simulink model "sim_tnse_2024_pos_ctrl"  (R2020a)
settings: Solver=ode4  StartTime=0.0  StopTime=30.0  FixedStep=0.01  RelTol=1e-3
values from neighbouring files (symbols this model uses):
  alfa_theta = 20    [init_tnse_2024_pos_ctrl.m]
  c1 = diag( [ 150.0, 120.0, 120.0 ] )    [init_tnse_2024_pos_ctrl.m]
  c1_diff_sigma_bar_v = diag([25; 30; 20])    [init_tnse_2024_pos_ctrl.m]
  c1v = diag([5.8; 6.5; 6.5])    [init_tnse_2024_pos_ctrl.m]
  c2 = diag( [ 80.0, 50.0, 50.0 ] )    [init_tnse_2024_pos_ctrl.m]
  c2_diff_sigma_bar_v = diag([50; 50; 10])    [init_tnse_2024_pos_ctrl.m]
  c2v = diag([5.8; 6.5; 6.5])    [init_tnse_2024_pos_ctrl.m]
  c3_diff_sigma_bar_v = diag([15; 15; 10])    [init_tnse_2024_pos_ctrl.m]
  c3v = diag([4.8; 6.4; 6.0])    [init_tnse_2024_pos_ctrl.m]
  dp_aa_t = 0.2 * ones(3, 5) + ( 1.0 - 0.2 ) * rand(3, 5)    [init_tnse_2024_pos_ctrl.m]
  dp_ff_t = [ 0.4 * ones(1, 5) + ( 1.0 - 0.4 ) * rand(1, 5);                      0.4 * ones(1, 5) + ( 1.0 - 0.4 ) * rand(1, 5);                      0.2 * ones(1, 5) + ( 0.6 - 0.2 ) * rand(1, 5) ]    [init_tnse_2024_pos_ctrl.m]
  dp_phi_t = ( - pi / 2 ) * ones(3, 5) + ( pi / 2 - ( - pi / 2 ) ) * rand(3, 5)    [init_tnse_2024_pos_ctrl.m]
  eps0 = [0.05; 0.01; 0.01]    [init_tnse_2024_pos_ctrl.m]
  etai_0 = zeros(3,5)    [init_tnse_2024_pos_ctrl.m]
  kai0 = [15; 10; 10]    [init_tnse_2024_pos_ctrl.m]
  kai_1_t = 0.02    [init_tnse_2024_pos_ctrl.m]
  kai_3_t = 0.1    [init_tnse_2024_pos_ctrl.m]
  ksii_0 = zeros(3,5)    [init_tnse_2024_pos_ctrl.m]
  lam0 = [15; 10; 10]    [init_tnse_2024_pos_ctrl.m]
  Lamd_diff_sigma_bar_v = 0.5    [init_tnse_2024_pos_ctrl.m]
  mass_i = zeros(1,NF)    [init_tnse_2024_pos_ctrl.m]
  Mii = diag([1;0;0;0;1])    [init_tnse_2024_pos_ctrl.m]
  pos0 = zeros(3, 1)    [init_tnse_2024_pos_ctrl.m]
  PZ0 = P0(3)    [init_tnse_2024_pos_ctrl.m]
  PZ1 = 10    [init_tnse_2024_pos_ctrl.m]
  Qci_init = repmat([1;0;0;0],1,NF)    [init_tnse_2024_pos_ctrl.m]
  R0 = 4    [init_tnse_2024_pos_ctrl.m]
  R1 = 8    [init_tnse_2024_pos_ctrl.m]
  Rx2 = 10    [init_tnse_2024_pos_ctrl.m]
  Ry2 = 6    [init_tnse_2024_pos_ctrl.m]
  Rz2 = 4    [init_tnse_2024_pos_ctrl.m]
  sat_sr_low = [-30, -30, -30]    [init_tnse_2024_pos_ctrl.m]
  sat_sr_up = [30, 30, 30]    [init_tnse_2024_pos_ctrl.m]
  T0 = 0    [init_tnse_2024_pos_ctrl.m]
  T1 = tseq1    (= 10)    [init_tnse_2024_pos_ctrl.m]
  T12 = tseq1 + tseq12    (= 20)    [init_tnse_2024_pos_ctrl.m]
  T2 = tseq1 + tseq12 + tseq2    (= 30)    [init_tnse_2024_pos_ctrl.m]
  theta0 = ( 2 / 5 ) * pi    (= 1.25663706144)    [init_tnse_2024_pos_ctrl.m]
  vel0 = zeros(3, 1)    [init_tnse_2024_pos_ctrl.m]
  Wij = [0,0,1,0,0;              0,0,1,1,0;              1,0,0,0,1;              0,1,1,0,0;              0,0,1,0,0]    [init_tnse_2024_pos_ctrl.m]
  X1 = 8    [init_tnse_2024_pos_ctrl.m]
  X2 = 2    [init_tnse_2024_pos_ctrl.m]
  X3 = 3    [init_tnse_2024_pos_ctrl.m]
  Y1 = 10    [init_tnse_2024_pos_ctrl.m]
  Y2 = 2    [init_tnse_2024_pos_ctrl.m]
  Y3 = 4    [init_tnse_2024_pos_ctrl.m]
  Z1 = 4    [init_tnse_2024_pos_ctrl.m]
  Z2 = -6    [init_tnse_2024_pos_ctrl.m]
  Z3 = 2    [init_tnse_2024_pos_ctrl.m]
  zeta_diff_sigma_bar_v = 0.08    [init_tnse_2024_pos_ctrl.m]
undefined symbols (not defined in the file or in its folder): cal_frac_squ, p_alfav1, p_alfav2, q_alfav1, q_alfav2
(part 4 of 4)

== matlab function sim_tnse_2024_pos_ctrl/follower tracking error agent 1 ==
  data: ksi_track_err_1 output; delta_ksi_vec input; delta_eta_vec input; ksi_i_vec input; eta_i_vec input; ksi0 input; eta_track_err_1 output; eta0 input
function [ksi_track_err_1, eta_track_err_1]  = fcn(delta_ksi_vec, delta_eta_vec, ksi_i_vec, eta_i_vec, ksi0, eta0)
%%%% 计算跟随者节点1号位置/速度跟踪误差
eta_track_err_1 = eta_i_vec(:,1) - delta_eta_vec(:,1) - eta0;
ksi_track_err_1 = ksi_i_vec(:,1) - delta_ksi_vec(:,1) - ksi0;

== matlab function sim_tnse_2024_pos_ctrl/follower tracking error agent 2 ==
  data: ksi_track_err_2 output; delta_ksi_vec input; delta_eta_vec input; ksi_i_vec input; eta_i_vec input; ksi0 input; eta_track_err_2 output; eta0 input
function [ksi_track_err_2, eta_track_err_2]  = fcn(delta_ksi_vec, delta_eta_vec, ksi_i_vec, eta_i_vec, ksi0, eta0)
%%%% 计算跟随者节点2号位置/速度跟踪误差
eta_track_err_2 = eta_i_vec(:,2) - delta_eta_vec(:,2) - eta0;
ksi_track_err_2 = ksi_i_vec(:,2) - delta_ksi_vec(:,2) - ksi0;

== matlab function sim_tnse_2024_pos_ctrl/follower tracking error agent 3 ==
  data: ksi_track_err_3 output; delta_ksi_vec input; delta_eta_vec input; ksi_i_vec input; eta_i_vec input; ksi0 input; eta_track_err_3 output; eta0 input
function [ksi_track_err_3, eta_track_err_3]  = fcn(delta_ksi_vec, delta_eta_vec, ksi_i_vec, eta_i_vec, ksi0, eta0)
%%%% 计算跟随者节点3号位置/速度跟踪误差
eta_track_err_3 = eta_i_vec(:,3) - delta_eta_vec(:,3) - eta0;
ksi_track_err_3 = ksi_i_vec(:,3) - delta_ksi_vec(:,3) - ksi0;

== matlab function sim_tnse_2024_pos_ctrl/follower tracking error agent 4 ==
  data: ksi_track_err_4 output; delta_ksi_vec input; delta_eta_vec input; ksi_i_vec input; eta_i_vec input; ksi0 input; eta_track_err_4 output; eta0 input
function [ksi_track_err_4, eta_track_err_4]  = fcn(delta_ksi_vec, delta_eta_vec, ksi_i_vec, eta_i_vec, ksi0, eta0)
%%%% 计算跟随者节点4号位置/速度跟踪误差
eta_track_err_4 = eta_i_vec(:,4) - delta_eta_vec(:,4) - eta0;
ksi_track_err_4 = ksi_i_vec(:,4) - delta_ksi_vec(:,4) - ksi0;

== matlab function sim_tnse_2024_pos_ctrl/follower tracking error agent 5 ==
  data: ksi_track_err_5 output; delta_ksi_vec input; delta_eta_vec input; ksi_i_vec input; eta_i_vec input; ksi0 input; eta_track_err_5 output; eta0 input
function [ksi_track_err_5, eta_track_err_5]  = fcn(delta_ksi_vec, delta_eta_vec, ksi_i_vec, eta_i_vec, ksi0, eta0)
%%%% 计算跟随者节点5号位置/速度跟踪误差
eta_track_err_5 = eta_i_vec(:,5) - delta_eta_vec(:,5) - eta0;
ksi_track_err_5 = ksi_i_vec(:,5) - delta_ksi_vec(:,5) - ksi0;

== matlab function sim_tnse_2024_pos_ctrl/combine follower eta ksi ==
  data: ksi_track_err_vec output; ksi_track_err_1 input; ksi_track_err_2 input; ksi_track_err_3 input; ksi_track_err_4 input; ksi_track_err_5 input; eta_track_err_vec output; eta_track_err_1 input; eta_track_err_2 input; eta_track_err_3 input; eta_track_err_4 input; eta_track_err_5 input
function [ksi_track_err_vec, eta_track_err_vec]  = fcn(ksi_track_err_1, ksi_track_err_2, ksi_track_err_3, ksi_track_err_4, ksi_track_err_5, ...
                                                                                    eta_track_err_1, eta_track_err_2, eta_track_err_3, eta_track_err_4, eta_track_err_5)
%%%% 合并所有跟随者的速度/位置向量
ksi_track_err_vec = [ksi_track_err_1(:), ksi_track_err_2(:), ksi_track_err_3(:), ksi_track_err_4(:), ksi_track_err_5(:)];
eta_track_err_vec = [eta_track_err_1(:), eta_track_err_2(:), eta_track_err_3(:), eta_track_err_4(:), eta_track_err_5(:)];

== matlab function sim_tnse_2024_pos_ctrl/depart Rc5 ==
  data: y output; x input
function y = fcn(x)
y = x(:,:,5);

end

== matlab function sim_tnse_2024_pos_ctrl/depart Rc1 ==
  data: y output; x input
function y = fcn(x)
y = x(:,:,1);

end

== matlab function sim_tnse_2024_pos_ctrl/depart Rc2 ==
  data: y output; x input
function y = fcn(x)
y = x(:,:,2);

end

== matlab function sim_tnse_2024_pos_ctrl/depart Rc3 ==
  data: y output; x input
function y = fcn(x)
y = x(:,:,3);

end

== matlab function sim_tnse_2024_pos_ctrl/depart Rc4 ==
  data: y output; x input
function y = fcn(x)
y = x(:,:,4);

end

== matlab function sim_tnse_2024_pos_ctrl/combine rho_hat ==
  data: rho_hat_1 input; rho_hat_vec output; rho_hat_2 input; rho_hat_3 input; rho_hat_4 input; rho_hat_5 input
function rho_hat_vec  = fcn(rho_hat_1, rho_hat_2, rho_hat_3, rho_hat_4, rho_hat_5)
%%%% 合并领导者加速度分布式观测器
rho_hat_vec = zeros(3,5);
rho_hat_vec(:,1) = rho_hat_1(:);
rho_hat_vec(:,2) = rho_hat_2(:);
rho_hat_vec(:,3) = rho_hat_3(:);
rho_hat_vec(:,4) = rho_hat_4(:);
rho_hat_vec(:,5) = rho_hat_5(:);

== matlab function sim_tnse_2024_pos_ctrl/rho_hat agent 1 ==
  data: lam0 input; rho_hat_1 output; sigmai_vec input
function rho_hat_1 = fcn(lam0, sigmai_vec)
%%%% 领导者加速度分布式观测器
iiuav = 1;
rho_hat_1 = lam0(:) .* tanh( sigmai_vec(:,iiuav) );

== matlab function sim_tnse_2024_pos_ctrl/rho_hat agent 2 ==
  data: lam0 input; rho_hat_2 output; sigmai_vec input
function rho_hat_2 = fcn(lam0, sigmai_vec)
%%%% 领导者加速度分布式观测器
iiuav = 2;
rho_hat_2 = lam0(:) .* tanh( sigmai_vec(:,iiuav) );

== matlab function sim_tnse_2024_pos_ctrl/rho_hat agent 3 ==
  data: lam0 input; rho_hat_3 output; sigmai_vec input
function rho_hat_3 = fcn(lam0, sigmai_vec)
%%%% 领导者加速度分布式观测器
iiuav = 3;
rho_hat_3 = lam0(:) .* tanh( sigmai_vec(:,iiuav) );

== matlab function sim_tnse_2024_pos_ctrl/rho_hat agent 4 ==
  data: lam0 input; rho_hat_4 output; sigmai_vec input
function rho_hat_4 = fcn(lam0, sigmai_vec)
%%%% 领导者加速度分布式观测器
iiuav = 4;
rho_hat_4 = lam0(:) .* tanh( sigmai_vec(:,iiuav) );

== matlab function sim_tnse_2024_pos_ctrl/rho_hat agent 5 ==
  data: lam0 input; rho_hat_5 output; sigmai_vec input
function rho_hat_5 = fcn(lam0, sigmai_vec)
%%%% 领导者加速度分布式观测器
iiuav = 5;
rho_hat_5 = lam0(:) .* tanh( sigmai_vec(:,iiuav) );

== matlab function sim_tnse_2024_pos_ctrl/cal si agent 1 ==
  data: Wij input; Mii input; si_1 output; delta_ksi_vec input; ksi0 input; ksi_i_vec input; ksi_d_est_vec input
function si_1 = fcn(Wij, Mii, delta_ksi_vec, ksi0, ksi_i_vec, ksi_d_est_vec)
%%%% 计算位置误差面
iiuav = 1;
si_1 = Mii(iiuav, iiuav) * ( ksi_i_vec(:,iiuav) - ksi0(:) - delta_ksi_vec(:,iiuav) ) ...
            + Mii(iiuav, iiuav) * ( ksi_d_est_vec(:,iiuav) - ksi0(:) );
for jjuav = 1:5
    si_1 = si_1 + Wij(iiuav, jjuav) * ( ( ksi_i_vec(:,iiuav) - delta_ksi_vec(:,iiuav) ) - ( ksi_i_vec(:,jjuav) - delta_ksi_vec(:,jjuav) ) ) ...
                        + Wij(iiuav, jjuav) * ( ksi_d_est_vec(:,iiuav) - ksi_d_est_vec(:,jjuav) );
end

== matlab function sim_tnse_2024_pos_ctrl/generate translational disturbance agent 1 ==
  data: dp_aa_t input; dp_ff_t input; dp_phi_t input; dp_1 output; t input
function dp_1 = fcn(dp_aa_t, dp_ff_t, dp_phi_t, t)
%%%% 平移动力学方程中的扰动项设置
epsil_t = zeros(3, 1);

for kk = 1:5
    epsil_t = epsil_t + dp_aa_t(:, kk) .* sin( 2 * pi * dp_ff_t(:, kk) * t + dp_phi_t(:, kk) );
end

dp_1 = [ epsil_t(1) + 1.6 * sin( 0.4 * t ) + 2.0 * cos( 0.5 * t ) + 1.4 * sin( 0.7 * t ) ...
                + 4 * exp( -0.1 * t ) * sin( 0.8 * t ) + 3 / ( 1 + exp( -0.2 * ( t - 15 ) ) ); ...
                epsil_t(2) + 1.2 * sin( 0.2 * t ) + 3 * cos( 0.4 * t ) + 0.8 * sin( 0.6 * t ) ...
                + 2 * exp( -0.15 * t ) * cos( 1.2 * t ) + 3 / ( 1 + exp( -0.3 * ( t - 25 ) ) ); ...
                epsil_t(3) + 1.8 * sin( 0.2 * t ) + 1.6 * sin( 0.3 * t ) + 1.6 * cos( 0.4 * t ) ...
                + 4 * exp( -0.05 * t ) * sin( 0.5 * t + pi / 4 ) + 3 / ( 1 + exp( -0.5 * ( t - 20 ) ) ) ];

== matlab function sim_tnse_2024_pos_ctrl/update dpsy psy agent 1 ==
  data: Wij input; Mii input; d_2_psy_1 output; delta_ksi_vec input; delta_eta_vec input; ksi_i_vec input; eta_i_vec input; ksi_d_est_vec input; eta_d_est_vec input
function d_2_psy_1 = fcn(Wij, Mii, delta_ksi_vec, delta_eta_vec, ksi_i_vec, eta_i_vec, ksi_d_est_vec, eta_d_est_vec)
%%%% 计算集群构型估计二阶导数
iiuav = 1;
err_v_est = Mii(iiuav, iiuav) * ( eta_d_est_vec(:,iiuav) - ( eta_i_vec(:,iiuav) - delta_eta_vec(:,iiuav) ) );
err_p_est = Mii(iiuav, iiuav) * ( ksi_d_est_vec(:,iiuav) - ( ksi_i_vec(:,iiuav) - delta_ksi_vec(:,iiuav) ) );
for jjuav = 1:5
    err_v_est = err_v_est + Wij(iiuav, jjuav) * ( ( eta_d_est_vec(:,iiuav) - ( eta_i_vec(:,iiuav) - delta_eta_vec(:,iiuav) ) ) ...
                                                                                - ( eta_d_est_vec(:,jjuav) - ( eta_i_vec(:,jjuav) - delta_eta_vec(:,jjuav) ) ) );
    err_p_est = err_p_est + Wij(iiuav, jjuav) * ( ( ksi_d_est_vec(:,iiuav) - ( ksi_i_vec(:,iiuav) - delta_ksi_vec(:,iiuav) ) ) ...
                                                                                - ( ksi_d_est_vec(:,jjuav) - ( ksi_i_vec(:,jjuav) - delta_ksi_vec(:,jjuav) ) ) );
end
d_2_psy_1 = -err_v_est(:) - err_p_est(:);

== matlab function sim_tnse_2024_pos_ctrl/cal si agent 3 ==
  data: Wij input; Mii input; si_3 output; delta_ksi_vec input; ksi0 input; ksi_i_vec input; ksi_d_est_vec input
function si_3 = fcn(Wij, Mii, delta_ksi_vec, ksi0, ksi_i_vec, ksi_d_est_vec)
%%%% 计算位置误差面
iiuav = 3;
si_3 = Mii(iiuav, iiuav) * ( ksi_i_vec(:,iiuav) - ksi0(:) - delta_ksi_vec(:,iiuav) ) ...
            + Mii(iiuav, iiuav) * ( ksi_d_est_vec(:,iiuav) - ksi0(:) );
for jjuav = 1:5
    si_3 = si_3 + Wij(iiuav, jjuav) * ( ( ksi_i_vec(:,iiuav) - delta_ksi_vec(:,iiuav) ) - ( ksi_i_vec(:,jjuav) - delta_ksi_vec(:,jjuav) ) ) ...
                        + Wij(iiuav, jjuav) * ( ksi_d_est_vec(:,iiuav) - ksi_d_est_vec(:,jjuav) );
end

== matlab function sim_tnse_2024_pos_ctrl/cal si agent 4 ==
  data: Wij input; Mii input; si_4 output; delta_ksi_vec input; ksi0 input; ksi_i_vec input; ksi_d_est_vec input
function si_4 = fcn(Wij, Mii, delta_ksi_vec, ksi0, ksi_i_vec, ksi_d_est_vec)
%%%% 计算位置误差面
iiuav = 4;
si_4 = Mii(iiuav, iiuav) * ( ksi_i_vec(:,iiuav) - ksi0(:) - delta_ksi_vec(:,iiuav) ) ...
            + Mii(iiuav, iiuav) * ( ksi_d_est_vec(:,iiuav) - ksi0(:) );
for jjuav = 1:5
    si_4 = si_4 + Wij(iiuav, jjuav) * ( ( ksi_i_vec(:,iiuav) - delta_ksi_vec(:,iiuav) ) - ( ksi_i_vec(:,jjuav) - delta_ksi_vec(:,jjuav) ) ) ...
                        + Wij(iiuav, jjuav) * ( ksi_d_est_vec(:,iiuav) - ksi_d_est_vec(:,jjuav) );
end

== matlab function sim_tnse_2024_pos_ctrl/cal si agent 5 ==
  data: Wij input; Mii input; si_5 output; delta_ksi_vec input; ksi0 input; ksi_i_vec input; ksi_d_est_vec input
function si_5 = fcn(Wij, Mii, delta_ksi_vec, ksi0, ksi_i_vec, ksi_d_est_vec)
%%%% 计算位置误差面
iiuav = 5;
si_5 = Mii(iiuav, iiuav) * ( ksi_i_vec(:,iiuav) - ksi0(:) - delta_ksi_vec(:,iiuav) ) ...
            + Mii(iiuav, iiuav) * ( ksi_d_est_vec(:,iiuav) - ksi0(:) );
for jjuav = 1:5
    si_5 = si_5 + Wij(iiuav, jjuav) * ( ( ksi_i_vec(:,iiuav) - delta_ksi_vec(:,iiuav) ) - ( ksi_i_vec(:,jjuav) - delta_ksi_vec(:,jjuav) ) ) ...
                        + Wij(iiuav, jjuav) * ( ksi_d_est_vec(:,iiuav) - ksi_d_est_vec(:,jjuav) );
end

== matlab function sim_tnse_2024_pos_ctrl/cal ri agent 2 ==
  data: Wij input; Mii input; delta_eta_vec input; ri_2 output; eta0 input; eta_i_vec input; eta_d_est_vec input
function ri_2 = fcn(Wij, Mii, delta_eta_vec, eta0, eta_i_vec, eta_d_est_vec)
%%%% 计算速度误差面
iiuav = 2;
ri_2 = Mii(iiuav, iiuav) * ( eta_i_vec(:,iiuav) - eta0(:) - delta_eta_vec(:,iiuav) ) ...
            + Mii(iiuav, iiuav) * ( eta_d_est_vec(:,iiuav) - eta0(:) );
for jjuav = 1:5
    ri_2 = ri_2 + Wij(iiuav, jjuav) * ( ( eta_i_vec(:,iiuav) - delta_eta_vec(:,iiuav) ) - ( eta_i_vec(:,jjuav) - delta_eta_vec(:,jjuav) ) ) ...
                        + Wij(iiuav, jjuav) * ( eta_d_est_vec(:,iiuav) - eta_d_est_vec(:,jjuav) );
end

== matlab function sim_tnse_2024_pos_ctrl/combine d_psy ==
  data: d_psy_1 input; d_psy_2 input; d_psy_3 input; d_psy_4 input; d_psy_5 input; d_psy_vec output
function d_psy_vec  = fcn(d_psy_1, d_psy_2, d_psy_3, d_psy_4, d_psy_5)
%%%% 合并集群构型估计导数
d_psy_vec = zeros(3,5);
d_psy_vec(:,1) = d_psy_1(:);
d_psy_vec(:,2) = d_psy_2(:);
d_psy_vec(:,3) = d_psy_3(:);
d_psy_vec(:,4) = d_psy_4(:);
d_psy_vec(:,5) = d_psy_5(:);

== matlab function sim_tnse_2024_pos_ctrl/combine psy ==
  data: psy_1 input; psy_2 input; psy_3 input; psy_4 input; psy_5 input; psy_vec output
function psy_vec  = fcn(psy_1, psy_2, psy_3, psy_4, psy_5)
%%%% 合并集群构型估计量
psy_vec = zeros(3,5);
psy_vec(:,1) = psy_1(:);
psy_vec(:,2) = psy_2(:);
psy_vec(:,3) = psy_3(:);
psy_vec(:,4) = psy_4(:);
psy_vec(:,5) = psy_5(:);

== matlab function sim_tnse_2024_pos_ctrl/cal eta_d_est ksi_d_est ==
  data: d_psy_vec input; psy_vec input; eta_d_est_vec output; eta_i_vec input; ksi_i_vec input; ksi_d_est_vec output
function [eta_d_est_vec, ksi_d_est_vec] = fcn(d_psy_vec, psy_vec, eta_i_vec, ksi_i_vec)
%%%% 计算跟随者期望速度/位置
eta_d_est_vec = zeros(3,5);
ksi_d_est_vec = zeros(3,5);
for iiuav = 1:5
    eta_d_est_vec(:,iiuav) = eta_i_vec(:,iiuav) + d_psy_vec(:,iiuav);
    ksi_d_est_vec(:,iiuav) = ksi_i_vec(:,iiuav) + psy_vec(:,iiuav);
end

== matlab function sim_tnse_2024_pos_ctrl/generate translational disturbance agent 2 ==
  data: dp_aa_t input; dp_ff_t input; dp_phi_t input; dp_2 output; t input
function dp_2 = fcn(dp_aa_t, dp_ff_t, dp_phi_t, t)
%%%% 平移动力学方程中的扰动项设置
epsil_t = zeros(3, 1);

for kk = 1:5
    epsil_t = epsil_t + dp_aa_t(:, kk) .* sin( 2 * pi * dp_ff_t(:, kk) * t + dp_phi_t(:, kk) );
end

dp_2 = [ epsil_t(1) + 1.6 * sin( 0.2 * t ) + 2.0 * cos( 0.3 * t ) + 1.4 * sin( 0.5 * t ) ...
                + 4 * exp( -0.1 * t ) * sin( 0.5 * t ) + 3 / ( 1 + exp( -0.2 * ( t - 15 ) ) ); ...
                epsil_t(2) + 1.2 * sin( 0.1 * t ) + 3 * cos( 0.2 * t ) + 0.8 * sin( 0.4 * t ) ...
                + 2 * exp( -0.15 * t ) * cos( 0.6 * t ) + 3 / ( 1 + exp( -0.3 * ( t - 25 ) ) ); ...
                epsil_t(3) + 1.8 * sin( 0.1 * t ) + 1.6 * sin( 0.2 * t ) + 1.6 * cos( 0.3 * t ) ...
                + 4 * exp( -0.05 * t ) * sin( 0.4 * t + pi / 4 ) + 3 / ( 1 + exp( -0.5 * ( t - 20 ) ) ) ];

== matlab function sim_tnse_2024_pos_ctrl/cal ri agent 3 ==
  data: Wij input; Mii input; delta_eta_vec input; ri_3 output; eta0 input; eta_i_vec input; eta_d_est_vec input
function ri_3 = fcn(Wij, Mii, delta_eta_vec, eta0, eta_i_vec, eta_d_est_vec)
%%%% 计算速度误差面
iiuav = 3;
ri_3 = Mii(iiuav, iiuav) * ( eta_i_vec(:,iiuav) - eta0(:) - delta_eta_vec(:,iiuav) ) ...
            + Mii(iiuav, iiuav) * ( eta_d_est_vec(:,iiuav) - eta0(:) );
for jjuav = 1:5
    ri_3 = ri_3 + Wij(iiuav, jjuav) * ( ( eta_i_vec(:,iiuav) - delta_eta_vec(:,iiuav) ) - ( eta_i_vec(:,jjuav) - delta_eta_vec(:,jjuav) ) ) ...
                        + Wij(iiuav, jjuav) * ( eta_d_est_vec(:,iiuav) - eta_d_est_vec(:,jjuav) );
end

== matlab function sim_tnse_2024_pos_ctrl/cal ri agent 4 ==
  data: Wij input; Mii input; delta_eta_vec input; ri_4 output; eta0 input; eta_i_vec input; eta_d_est_vec input
function ri_4 = fcn(Wij, Mii, delta_eta_vec, eta0, eta_i_vec, eta_d_est_vec)
%%%% 计算速度误差面
iiuav = 4;
ri_4 = Mii(iiuav, iiuav) * ( eta_i_vec(:,iiuav) - eta0(:) - delta_eta_vec(:,iiuav) ) ...
            + Mii(iiuav, iiuav) * ( eta_d_est_vec(:,iiuav) - eta0(:) );
for jjuav = 1:5
    ri_4 = ri_4 + Wij(iiuav, jjuav) * ( ( eta_i_vec(:,iiuav) - delta_eta_vec(:,iiuav) ) - ( eta_i_vec(:,jjuav) - delta_eta_vec(:,jjuav) ) ) ...
                        + Wij(iiuav, jjuav) * ( eta_d_est_vec(:,iiuav) - eta_d_est_vec(:,jjuav) );
end

== matlab function sim_tnse_2024_pos_ctrl/cal ri agent 5 ==
  data: Wij input; Mii input; delta_eta_vec input; ri_5 output; eta0 input; eta_i_vec input; eta_d_est_vec input
function ri_5 = fcn(Wij, Mii, delta_eta_vec, eta0, eta_i_vec, eta_d_est_vec)
%%%% 计算速度误差面
iiuav = 5;
ri_5 = Mii(iiuav, iiuav) * ( eta_i_vec(:,iiuav) - eta0(:) - delta_eta_vec(:,iiuav) ) ...
            + Mii(iiuav, iiuav) * ( eta_d_est_vec(:,iiuav) - eta0(:) );
for jjuav = 1:5
    ri_5 = ri_5 + Wij(iiuav, jjuav) * ( ( eta_i_vec(:,iiuav) - delta_eta_vec(:,iiuav) ) - ( eta_i_vec(:,jjuav) - delta_eta_vec(:,jjuav) ) ) ...
                        + Wij(iiuav, jjuav) * ( eta_d_est_vec(:,iiuav) - eta_d_est_vec(:,jjuav) );
end

== matlab function sim_tnse_2024_pos_ctrl/combine si ==
  data: si_1 input; si_2 input; si_3 input; si_4 input; si_5 input; si_vec output
function si_vec  = fcn(si_1, si_2, si_3, si_4, si_5)
%%%% 合并位置跟踪误差
si_vec = zeros(3,5);
si_vec(:,1) = si_1(:);
si_vec(:,2) = si_2(:);
si_vec(:,3) = si_3(:);
si_vec(:,4) = si_4(:);
si_vec(:,5) = si_5(:);

== matlab function sim_tnse_2024_pos_ctrl/cal ri agent 1 ==
  data: Wij input; Mii input; delta_eta_vec input; ri_1 output; eta0 input; eta_i_vec input; eta_d_est_vec input
function ri_1 = fcn(Wij, Mii, delta_eta_vec, eta0, eta_i_vec, eta_d_est_vec)
%%%% 计算速度误差面
iiuav = 1;
ri_1 = Mii(iiuav, iiuav) * ( eta_i_vec(:,iiuav) - eta0(:) - delta_eta_vec(:,iiuav) ) ...
            + Mii(iiuav, iiuav) * ( eta_d_est_vec(:,iiuav) - eta0(:) );
for jjuav = 1:5
    ri_1 = ri_1 + Wij(iiuav, jjuav) * ( ( eta_i_vec(:,iiuav) - delta_eta_vec(:,iiuav) ) - ( eta_i_vec(:,jjuav) - delta_eta_vec(:,jjuav) ) ) ...
                        + Wij(iiuav, jjuav) * ( eta_d_est_vec(:,iiuav) - eta_d_est_vec(:,jjuav) );
end

== matlab function sim_tnse_2024_pos_ctrl/combine ri ==
  data: ri_1 input; ri_2 input; ri_3 input; ri_4 input; ri_5 input; ri_vec output
function ri_vec  = fcn(ri_1, ri_2, ri_3, ri_4, ri_5)
%%%% 合并速度跟踪误差
ri_vec = zeros(3,5);
ri_vec(:,1) = ri_1(:);
ri_vec(:,2) = ri_2(:);
ri_vec(:,3) = ri_3(:);
ri_vec(:,4) = ri_4(:);
ri_vec(:,5) = ri_5(:);

== matlab function sim_tnse_2024_pos_ctrl/leader control input ==
  data: t input; u0 output; T1 input; T2 input; R0 input; R1 input; Rx2 input; Ry2 input; Rz2 input
function u0  = fcn(t, T1, T2, R0, R1, Rx2, Ry2, Rz2)
%%%% 给出领导者参考加速度控制输入
u0 = zeros(3, 1);

if t <= ( T1 + 1e-05 )
    u0(1, 1) = - ( 4 * pi * sin( ( 2 * pi * ( t - 0 ) ) / ( 0 - T1 ) ) * ( R0 - R1 ) ) / ( ( 0 - T1 ) ^ 2 ) ...
                        - ( 4 * ( pi ^ 2 ) * cos( ( 2 * pi * ( t - 0 ) ) / ( 0 - T1 ) ) ...
                        * ( R0 + ( ( R0 - R1 ) * ( t - 0 ) ) / ( 0 - T1 ) ) ) / ( ( 0 - T1 ) ^ 2 );
    u0(2, 1) = ( 4 * pi * cos( ( 2 * pi * ( t - 0 ) ) / ( 0 - T1 ) ) * ( R0 - R1 ) ) / ( ( 0 - T1 ) ^ 2 ) ...
                        - ( 4 * ( pi ^ 2 ) * sin( ( 2 * pi * ( t - 0 ) ) / ( 0 - T1 ) ) ...
                        * ( R0 + ( ( R0 - R1 ) * ( t - 0 ) ) / ( 0 - T1 ) ) ) / ( ( 0 - T1 ) ^ 2 );
    u0(3, 1) = 0;
else
    u0(1, 1) = ( 4 * Rx2 * ( pi ^ 2 ) * cos( ( 2 * pi * ( t - T1 ) ) / ( T1 - T2 ) ) ) / ( ( T1 - T2 ) ^ 2 );
    u0(2, 1) = - ( 16 * Ry2 * ( pi ^ 2 ) * sin( ( 4 * pi * ( t - T1 ) ) / ( T1 - T2 ) ) ) / ( ( T1 - T2 ) ^ 2 );
    u0(3, 1) = ( 16 * Rz2 * ( pi ^ 2 ) * sin( ( 4 * pi * ( t - T1 ) ) / ( T1 - T2 ) ) ) / ( ( T1 - T2 ) ^ 2 );
end

== matlab function sim_tnse_2024_pos_ctrl/process velocity ==
  data: T0 input; T1 input; T2 input; PZ0 input; PZ1 input; R0 input; R1 input; Rx2 input; Ry2 input; Rz2 input; t input; V_init_out output
function V_init_out = fcn(T0, T1, T2, PZ0, PZ1, R0, R1, Rx2, Ry2, Rz2, t)
V_init_out = zeros(3, 1);
if t < T1 + 1e-05
    V_init_out(1, 1) = ( cos( ( 2 * pi * ( t - T0 ) ) / ( T0 - T1 ) ) * ( R0 - R1 ) ) / ( T0 - T1 ) ...
                                    - ( 2 * pi * sin( ( 2 * pi * ( t - T0 ) ) / ( T0 - T1 ) ) * ( R0 + ( ( R0 - R1 ) * ( t - T0 ) ) / ( T0 - T1 ) ) ) / ( T0 - T1 );
    V_init_out(2, 1) = ( sin( ( 2 * pi * ( t - T0 ) ) / ( T0 - T1 ) ) * ( R0 - R1 ) ) / ( T0 - T1 ) ...
                                    + ( 2 * pi * cos( ( 2 * pi * ( t - T0 ) ) / ( T0 - T1 ) ) * ( R0 + ( ( R0 - R1 ) * ( t - T0 ) ) / ( T0 - T1 ) ) ) / ( T0 - T1 );
    V_init_out(3, 1) = ( PZ0 - PZ1 ) / ( T0 - T1 );
else
    V_init_out(1, 1) = ( 2 * Rx2 * pi * sin( ( 2 * pi * ( t - T1 ) ) / ( T1 - T2 ) ) ) / ( T1 - T2 );
    V_init_out(2, 1) = ( 4 * Ry2 * pi * cos( ( 4 * pi * ( t - T1 ) ) / ( T1 - T2 ) ) ) / ( T1 - T2 );
    V_init_out(3, 1) = - ( 4 * Rz2 * pi * cos( ( 4 * pi * ( t - T1 ) ) / ( T1 - T2 ) ) ) / ( T1 - T2 );
end

== matlab function sim_tnse_2024_pos_ctrl/generate translational disturbance agent 3 ==
  data: dp_aa_t input; dp_ff_t input; dp_phi_t input; dp_3 output; t input
function dp_3 = fcn(dp_aa_t, dp_ff_t, dp_phi_t, t)
%%%% 平移动力学方程中的扰动项设置
epsil_t = zeros(3, 1);

for kk = 1:5
    epsil_t = epsil_t + dp_aa_t(:, kk) .* sin( 2 * pi * dp_ff_t(:, kk) * t + dp_phi_t(:, kk) );
end

dp_3 = [ epsil_t(1) + 1.6 * sin( 0.2 * t ) + 2.0 * cos( 0.3 * t ) + 1.4 * sin( 0.5 * t ) ...
                + 4 * exp( -0.1 * t ) * sin( 0.5 * t ) + 3 / ( 1 + exp( -0.2 * ( t - 15 ) ) ); ...
                epsil_t(2) + 1.2 * sin( 0.1 * t ) + 3 * cos( 0.2 * t ) + 0.8 * sin( 0.4 * t ) ...
                + 2 * exp( -0.15 * t ) * cos( 0.6 * t ) + 3 / ( 1 + exp( -0.3 * ( t - 25 ) ) ); ...
                epsil_t(3) + 1.8 * sin( 0.1 * t ) + 1.6 * sin( 0.2 * t ) + 1.6 * cos( 0.3 * t ) ...
                + 4 * exp( -0.05 * t ) * sin( 0.4 * t + pi / 4 ) + 3 / ( 1 + exp( -0.5 * ( t - 20 ) ) ) ];

== matlab function sim_tnse_2024_pos_ctrl/set desire formation configuration ==
  data: X1 input; X2 input; X3 input; Y1 input; Y2 input; Y3 input; Z1 input; Z2 input; Z3 input; theta0 input; kai_1_t input; kai_3_t input; T1 input; T12 input; t input; delta_ksi_vec output; delta_eta_vec output; d_delta_eta_vec output
function [delta_ksi_vec, delta_eta_vec, d_delta_eta_vec] = fcn(X1, X2, X3, Y1, Y2, Y3, Z1, Z2, Z3, ...
                                                                                                                theta0, kai_1_t, kai_3_t, T1, T12, t)
%%%% 计算跟随者期望速度分布式观测器误差
delta_ksi_vec = zeros(3, 5);
delta_eta_vec = zeros(3, 5);
d_delta_eta_vec = zeros(3, 5);
if t <= ( T1 + 1e-04 )
    exp_tmp = exp( -kai_1_t * t );
    delta_ksi_vec(:, 1) = [ X1 * cos( theta0 ) - X2 * exp_tmp; ...
                                            Y1 * sin( theta0 ) - Y2 * exp_tmp; ...
                                            Z1 - Z2 * exp_tmp ];
    delta_ksi_vec(:, 2) = [ - X1 * cos( theta0 ) + X2 * exp_tmp; ...
                                            Y1 * sin( theta0 ) - Y2 * exp_tmp; ...
                                            Z1 + Z2 * exp_tmp ];
    delta_ksi_vec(:, 3) = [ X1 - X2 * exp_tmp; ...
                                            Y2 * exp_tmp; ...
                                            ( 3 / 8 ) * Z1 + Z2 * exp_tmp ];
    delta_ksi_vec(:, 4) = [ - X1 * cos( theta0 ) + X2 * exp_tmp; ...
                                            - Y1 * sin( theta0 ) + Y2 * exp_tmp; ...
                                            Z1 + Z2 * exp_tmp ];
    delta_ksi_vec(:, 5) = [ X1 * cos( theta0 ) - X2 * exp_tmp; ...
                                            - Y1 * sin( theta0 ) + Y2 * exp_tmp; ...
                                            Z1 - Z2 * exp_tmp ];
    delta_eta_vec(:, 1) = [ kai_1_t * X2 * exp_tmp; kai_1_t * Y2 * exp_tmp; kai_1_t * Z2 * exp_tmp ];
    delta_eta_vec(:, 2) = [ - kai_1_t * X2 * exp_tmp; kai_1_t * Y2 * exp_tmp; - kai_1_t * Z2 * exp_tmp ];
    delta_eta_vec(:, 3) = [ kai_1_t * X2 * exp_tmp; - kai_1_t * Y2 * exp_tmp; - kai_1_t * Z2 * exp_tmp ];
    delta_eta_vec(:, 4) = [ - kai_1_t * X2 * exp_tmp; - kai_1_t * Y2 * exp_tmp; - kai_1_t * Z2 * exp_tmp ];
    delta_eta_vec(:, 5) = [ kai_1_t * X2 * exp_tmp; - kai_1_t * Y2 * exp_tmp; kai_1_t * Z2 * exp_tmp ];
    d_delta_eta_vec(:, 1) = [ - ( kai_1_t ^ 2 ) * X2 * exp_tmp; - ( kai_1_t ^ 2 ) * Y2 * exp_tmp; - ( kai_1_t ^ 2 ) * Z2 * exp_tmp ];
    d_delta_eta_vec(:, 2) = [ ( kai_1_t ^ 2 ) * X2 * exp_tmp; - ( kai_1_t ^ 2 ) * Y2 * exp_tmp; ( kai_1_t ^ 2 ) * Z2 * exp_tmp ];
    d_delta_eta_vec(:, 3) = [ - ( kai_1_t ^ 2 ) * X2 * exp_tmp; ( kai_1_t ^ 2 ) * Y2 * exp_tmp; ( kai_1_t ^ 2 ) * Z2 * exp_tmp ];
    d_delta_eta_vec(:, 4) = [ ( kai_1_t ^ 2 ) * X2 * exp_tmp; ( kai_1_t ^ 2 ) * Y2 * exp_tmp; ( kai_1_t ^ 2 ) * Z2 * exp_tmp ];
    d_delta_eta_vec(:, 5) = [ - ( kai_1_t ^ 2 ) * X2 * exp_tmp; ( kai_1_t ^ 2 ) * Y2 * exp_tmp; - ( kai_1_t ^ 2 ) * Z2 * exp_tmp ];
elseif t <= ( T12 + 1e-04 )
    delta_ksi_vec(:, 1) = [ X1 * cos( theta0 ) - X2; Y1 * sin( theta0 ) - Y2; Z1 - Z2 ];
    delta_ksi_vec(:, 2) = [ - X1 * cos( theta0 ) + X2; Y1 * sin( theta0 ) - Y2; Z1 + Z2 ];
    delta_ksi_vec(:, 3) = [ X1 - X2; 0; ( 3 / 8 ) * Z1 + Z2 ];
    delta_ksi_vec(:, 4) = [ - X1 * cos( theta0 ) + X2; - Y1 * sin( theta0 ) + Y2; Z1 + Z2 ];
    delta_ksi_vec(:, 5) = [ X1 * cos( theta0 ) - X2; - Y1 * sin( theta0 ) + Y2; Z1 - Z2 ];
else
    exp_tmp = 1 / ( 1 + exp( - kai_3_t * ( t - T12 - 5 ) ) );
    tmp_2 = exp( - kai_3_t * ( t - T12 - 5 ) ) / ( ( 1 + exp( - kai_3_t * ( t - T12 - 5 ) ) ) ^ 2 );
    delta_ksi_vec(:, 1) = [ X1 * cos( theta0 ) - X2 + X3 * exp_tmp; ...
                                            Y1 * sin( theta0 ) - Y2 + Y3 * exp_tmp; ...
                                            Z1 - Z2 + Z3 * exp_tmp ];
    delta_ksi_vec(:, 2) = [ - X1 * cos( theta0 ) + X2 - X3 * exp_tmp; ...
                                            Y1 * sin( theta0 ) - Y2 + Y3 * exp_tmp; ...
                                            Z1 + Z2 - Z3 * exp_tmp ];
    delta_ksi_vec(:, 3) = [ X1 - X2 + X3 * exp_tmp; ...
                                            - Y3 * exp_tmp; ...
                                            ( 3 / 8 ) * Z1 + Z2 - Z3 * exp_tmp ];
    delta_ksi_vec(:, 4) = [ - X1 * cos( theta0 ) + X2 - X3 * exp_tmp; ...
                                            - Y1 * sin( theta0 ) + Y2 - Y3 * exp_tmp; ...
                                            Z1 + Z2 - Z3 * exp_tmp ];
    delta_ksi_vec(:, 5) = [ X1 * cos( theta0 ) - X2 + X3 * exp_tmp; ...
                                            - Y1 * sin( theta0 ) + Y2 - Y3 * exp_tmp; ...
                                            Z1 - Z2 + Z3 * exp_tmp ];
    delta_eta_vec(:, 1) = [ kai_3_t * X3 * tmp_2; kai_3_t * Y3 * tmp_2; kai_3_t * Z3 * tmp_2 ];
    delta_eta_vec(:, 2) = [ - kai_3_t * X3 * tmp_2; kai_3_t * Y3 * tmp_2; kai_3_t * Z3 * tmp_2 ];
    delta_eta_vec(:, 3) = [ kai_3_t * X3 * tmp_2; - kai_3_t * Y3 * tmp_2; - kai_3_t * Z3 * tmp_2 ];
    delta_eta_vec(:, 4) = [ - kai_3_t * X3 * tmp_2; - kai_3_t * Y3 * tmp_2; - kai_3_t * Z3 * tmp_2 ];
    delta_eta_vec(:, 5) = [ kai_3_t * X3 * tmp_2; kai_3_t * Y3 * tmp_2; - kai_3_t * Z3 * tmp_2 ];
    d_delta_eta_vec(:, 1) = ( kai_3_t * ( 1 - exp( - kai_3_t * ( t - T12 - 5 ) ) ) * exp_tmp ) * delta_eta_vec(:, 1);
    d_delta_eta_vec(:, 2) = ( kai_3_t * ( 1 - exp( - kai_3_t * ( t - T12 - 5 ) ) ) * exp_tmp ) * delta_eta_vec(:, 2);
    d_delta_eta_vec(:, 3) = ( kai_3_t * ( 1 - exp( - kai_3_t * ( t - T12 - 5 ) ) ) * exp_tmp ) * delta_eta_vec(:, 3);
    d_delta_eta_vec(:, 4) = ( kai_3_t * ( 1 - exp( - kai_3_t * ( t - T12 - 5 ) ) ) * exp_tmp ) * delta_eta_vec(:, 4);
    d_delta_eta_vec(:, 5) = ( kai_3_t * ( 1 - exp( - kai_3_t * ( t - T12 - 5 ) ) ) * exp_tmp ) * delta_eta_vec(:, 5);
end

== matlab function sim_tnse_2024_pos_ctrl/cal virtual control sigma_v agent 1 ==
  data: c3v input; Ri input; ui_vec input; d_sigma_v_1 output; sigma_bar_v_vec input
function d_sigma_v_1 = fcn(c3v, Ri, ui_vec, sigma_bar_v_vec)
%%%% 计算扰动观测器中虚拟速度控制量sigma_v的微分方程

iiuav = 1;
g0 = 9.80663;
e3 = [0;0;1];
d_sigma_v_1 = -g0 * e3 + norm(ui_vec(:,iiuav), 2) * Ri(:,:,iiuav) * e3 + c3v * sigma_bar_v_vec(:,iiuav);

== matlab function sim_tnse_2024_pos_ctrl/cal virtual control sigma_v agent 2 ==
  data: c3v input; Ri input; ui_vec input; d_sigma_v_2 output; sigma_bar_v_vec input
function d_sigma_v_2 = fcn(c3v, Ri, ui_vec, sigma_bar_v_vec)
%%%% 计算扰动观测器中虚拟速度控制量sigma_v的微分方程

iiuav = 2;
g0 = 9.80663;
e3 = [0;0;1];
d_sigma_v_2 = -g0 * e3 + norm(ui_vec(:,iiuav), 2) * Ri(:,:,iiuav) * e3 + c3v * sigma_bar_v_vec(:,iiuav);
